simulink model "base_reference"  (R2019a)
settings: Solver=ode23tb  StartTime=0.0  StopTime=60  RelTol=1e-3
model workspace (MAT data in the model file):
  A_mu = 10
  AxlIxx = 62.3745166667
  AxlM = 160
  B_reff = 8.386
  BattCapInit = 26
  BattChargeMax = 32.5
  BattChrgMax = -80000
  BattDischrgMax = 80000
  BattTempBp = [243.1 253.1 263.1 273.1 283.1 298.1 313.1]
  BrkPrsMax = 5000000
  CapLUTBp = [0 0.01 0.02 0.03 0.04 0.05 0.06 0.07 0.08 0.09 0.1 0.11 ... (101 elements, 1x101)]
  CapSOCBp = [0 0.2 0.4 0.6 0.8 1]
  ChrgLmt_bpt = [1 1 1 1 1 1 1 1 0.7 0.35 0]
  Cps = 2
  Cz = 5565.2246438
  CzWhlAxl = 11490.971257
  DCT_Param : struct (value not decoded)
  DLCXref = [0 6 7 14 33.5 34 42 50 60]
  DLCYref = [0 0 -4.5 -4 -3.75 1.5 0.5 0 0]
  D_reff = 0.25826
  DischrgLmt_bpt = [0 0.35 0.7 1 1 1 1 1 1 1 1]
  Downshift_Speeds = [9.5625 12.9375 16.3125 19.6875 23.0625 26.4375 29.8125 33.1875 36.5625 39.9375 43.3125 46.6875 ... (28 elements, 4x7)]
  EV_current = 200
  EV_motion = [20 4 0.8]
  EV_sf = 2000
  Em = [2.8 3.228 3.284 3.361 3.408 3.427 3.472 3.477 3.493 3.504 3.516 3.528 ... (101 elements, 1x101)]
  EngRevLim = 7000
  F0z = [2886 2907]
  F0zWhlAxl = 2907
  Fs = 0
  Fv = 0.0025
  Hmax = 0.25
  Jcomp = 0.0227
  Ki = 251.3274
  Kisa = 346.6583
  Kp_d = 0.47149
  Kp_q = 0.52125
  Ksa = 85.4316
  Ksf = 1996.2651
  Kz = 52451.0065793
  KzWhlAxl = 138031.612078
  Ld = 0.0003752
  Ldq = [0.0003752 0.0004148]
  Lq = 0.0004148
  Mechanical = [0.0227 0.0025 0]
  MotMapEff = 0
  MotSpd = [0 1000 2000 2728.370453 3000 4000 5000 6000 7000 8000 9000 10000]
  MotTrq = [280 280 280 280 254.6479089 190.9859317 152.7887454 127.3239545 109.1348181 95.49296586 84.88263632 76.39437268]
  NCyl = 6
  Ndiff = 7.94
  Np = 2
  Ns = 96
  P = 4
  Pedal_Positions = [0.1 0.4 0.5 0.9]
  PolePairs = 4
  Pstd = 101325
  RInt = [0.008846 0.006389 0.004364 0.002031 0.001443 0.0005603 0.001028 0.009319 0.006554 0.004101 0.002563 0.001825 ... (42 elements, 7x6)]
  Rair = 287
  RegenBrkCutOff = [0 1]
  RegenBrkSpd_bpt = [5 9]
  Rm = 0.15
  Rs = 0.2
  SOC_bpt = [0 10 20 30 40 50 60 70 80 90 100]
  SUS : struct (value not decoded)
  T_eff_bp = [0 20 40 60 80 100 120 140 160 180 200 220 ... (15 elements, 1x15)]
  T_max = 120
  T_mtpa = [0 13.3131834767 26.6278836885 39.9456159322 53.2678926341 66.5962219318 79.9321062746 93.277041051 106.632513247 120.000000141]
  Tc = 0.02
  Trans : struct (value not decoded)
  Tstd = 293.15
  Upshift_Speeds = [12.9375 16.3125 19.6875 33 26.4375 29.8125 33.1875 52.5 39.9375 43.3125 46.6875 77.25 ... (28 elements, 4x7)]
  VEH : struct (value not decoded)
  V_o = 16.7
  V_xlow = 1
  Vd = 0.00346
  WH : struct (value not decoded)
  a = 1.4
  alpha_max = 1.5
  alpha_min = -1.5
  b = 1.8
  ba = 3.4029
  c_zo = 209651
  disk_abore = 0.05
  dt3D = 0.05
  efficiency_table = [85 85 85 85 85 85 85 85 85 85 85 85 ... (180 elements, 12x15)]
  epsilon = 0.1
  f_air = [0 0 0 0 0 0 0 0 0 0 0 0 ... (256 elements, 16x16)]
  f_co = [0 0 0 0 0 0 0 0 0 0 0 0 ... (256 elements, 16x16)]
  f_co2 = [0 0 0 0 0 0 0 0 0 0 0 0 ... (256 elements, 16x16)]
  f_eff = [352.135682859 352.135682859 320.724378192 303.655312657 295.930136708 291.240087194 291.240271258 291.240312459 291.240275452 291.240198499 291.240100781 291.240018769 ... (256 elements, 16x16)]
  f_fuel = [0 0 0 0 0 0 0 0 0 0 0 0 ... (256 elements, 16x16)]
  f_hc = [0 0 0 0 0 0 0 0 0 0 0 0 ... (256 elements, 16x16)]
  f_nox = [0 0 0 0 0 0 0 0 0 0 0 0 ... (256 elements, 16x16)]
  f_pm = [0 0 0 0 0 0 0 0 0 0 0 0 ... (256 elements, 16x16)]
  f_susp_axl_bp = [1 2]
  f_susp_dz_bp = [-0.325022776267 -0.315022776267 -0.305022776267 -0.205022776267 -0.105022776267 -0.00502277626717 0.0949772237328 0.194977223733 0.204977223733 0.214977223733]
  f_susp_dzdot_bp = [-3 -0.3 -0.2 -0.1 0 0.1 0.2 0.3 3]
  f_susp_fmz = [-144070.391448 -93629.24037 -75929.1118915 -20630.5828179 -15385.48216 -10140.3815021 -4895.28084414 349.819813785 -31916.3973792 18437.6709544 -83996.1993354 -33555.0482577 ... (43920 elements, 10x9x61x2x4)]
  f_susp_geom = [0 0 0 0 0 0 0 0 0 0 0 0 ... (3660 elements, 10x61x2x3)]
  f_susp_strgdelta_bp = [-0.523598775598 -0.506145483078 -0.488692190558 -0.471238898038 -0.453785605519 -0.436332312999 -0.418879020479 -0.401425727959 -0.383972435439 -0.366519142919 -0.349065850399 -0.331612557879 ... (61 elements, 1x61)]
  f_tbrake = [0 76.8593923996 105.140482948 131.533638111 157.926793274 176.658631717 176.65727296 176.656856686 176.656879077 176.657093756 176.657404516 176.65772406 ... (256 elements, 16x16)]
  f_tbrake_n_bpt = [0 649.519052838 912.419621844 1175.32019085 1438.22075986 1701.12132886 1964.02189787 2226.92246687 2489.82303588 2752.72360489 3015.62417389 3278.5247429 ... (16 elements, 1x16)]
  f_tbrake_t_bpt = [0 34.6410161514 61.0341713143 87.4273264773 113.82048164 140.213636803 166.606791966 192.999947129 219.393102292 245.786257455 272.179412618 298.572567781 ... (16 elements, 1x16)]
  f_texh = [766.752464599 766.752464599 786.17542386 801.679939032 884.591982581 910.574397722 910.571871054 910.570774534 910.570601632 910.570821151 910.571247242 910.571639815 ... (256 elements, 16x16)]
  f_twc_eff_co = [0.17 0.25 0.45 0.99 0.99 0.99 0.99]
  f_twc_eff_hc = [0.21 0.375 0.75 0.98 0.98 0.98 0.98]
  f_twc_eff_lam = [0.909090909 0.944055944 0.979020979 1 1.013986014 1.048951049 1.083916084]
  f_twc_eff_nox = [0.98 0.98 0.98 0.97 0.05 0.02 0]
  h = 0.134
  id_mtpa = [0 -0.114523352646 -0.457989076459 -1.03008464374 -1.83029075221 -2.85788367342 -4.11193850568 -5.59133329791 -7.29475400168 -9.22070020138]
  idq0 = [0 0]
  idq_limits = [-9.220699542 166.993501392 167.247872355]
  iq_mtpa = [0 18.5827440345 37.1633719111 55.7397734896 74.3098506185 92.871523015 111.422734008 129.961456105 148.485696337 166.993501356]
  lambda_pm = 0.1194
  mechanical = [0.0227 0.0025 0]
  mu_kinetic = 0.35
  numWheel = 4
  num_pads = 2
  omega_init = 0
  path : struct (value not decoded)
  pio = 220000
  power_max = 80000
  q_Fcx = 0
  q_Fz2 = 15.4
  q_Fzy = 0
  q_reo = 0.9974
  q_sx1 = -0.007764
  q_sx10 = 0.2824
  q_sx11 = 5.349
  q_sx12 = 0
  q_sx13 = 0
  q_sx14 = 0
  q_sx2 = 1.1915
  q_sx3 = 0.013948
  q_sx4 = 4.912
  q_sx5 = 1.02
  q_sx6 = 22.83
  q_sx7 = 0.7104
  q_sx8 = -0.023393
  q_sx9 = 0.6581
  q_sy1 = 0.00702
  q_sy2 = 0
  q_sy3 = 0.001515
  q_sy4 = 8.514e-05
  q_sy5 = 0
  q_sy6 = 0
  q_sy7 = 0.9008
  q_sy8 = -0.4089
  q_v1 = 0.0007742
  q_v2 = 0.04667
  r_Bx1 = 12.531
  r_Bx2 = 9.532
  r_Bx3 = 0
  r_By1 = 10.615
  r_By2 = 7.705
  r_By3 = 3.433e-06
  r_By4 = 0
  r_Cx1 = 1.019
  r_Cy1 = 1.0585
  r_Ex1 = -0.4487
  r_Ex2 = -0.4726
  r_Ey1 = 0.3132
  r_Ey2 = 7.63e-06
  r_Hx1 = 0.0002374
  r_Hy1 = 0.011646
  r_Hy2 = 7.63e-06
  r_Vy1 = 0.05654
  r_Vy2 = 7.63e-06
  r_Vy3 = 0
  r_Vy4 = 99.9
  r_Vy5 = 2
  r_Vy6 = 15.814
  r_o = 0.3135
  theta_init = 0
  torque_max = 280
  vehWidth = 2
  w = 1
  w_eff_bp = [0 1000 2000 2728.370453 3000 4000 5000 6000 7000 8000 9000 10000]
values from neighbouring files (symbols this model uses):
  VEH =     [PassVeh14DOF.mat]    (also in model2.mat; model_workspace_reference.mat)
undefined symbols (not defined in the file or in its folder): Disabled, Right
libraries: simulink x8, vehdynlibtire x8, vehdynlibsuspension x7, autolibutils x6, vehdynlibscenariocommon x5, sim3dlib x4, autolibmappedmotor x4, autolibshared x2, sharedtransform x2, vehdynlibviscommon x2, vehdynlibdriver x1, vehdynlibsteering x1
(part 3 of 8)

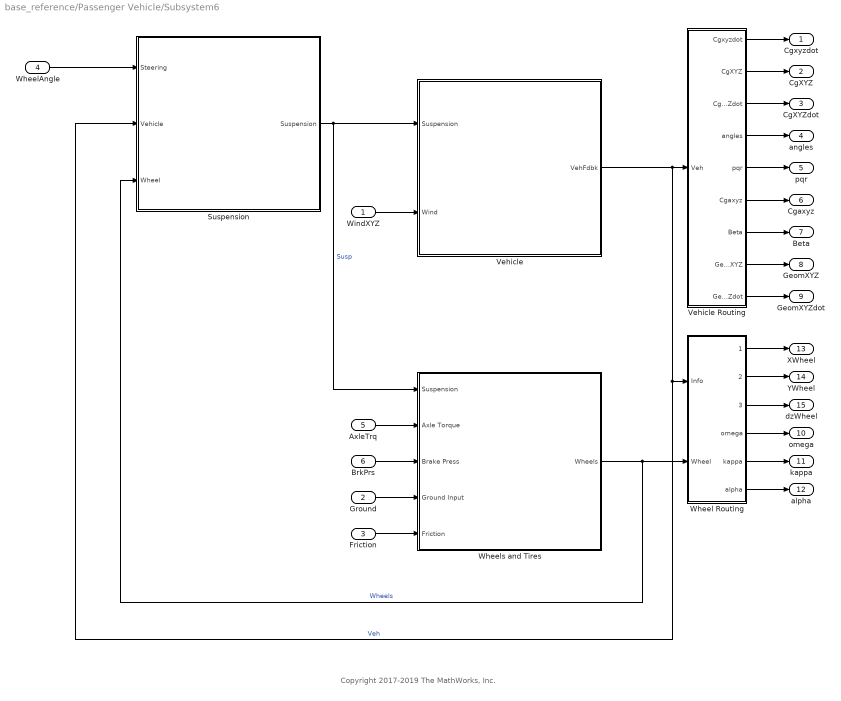
== system base_reference/Passenger Vehicle/Subsystem6 ==
  note: Copyright 2017-2019 The MathWorks, Inc.
  WindXYZ : Inport  Unit=m/s  PortDimensions=3
  Ground : Inport  Port=2  Unit=m  PortDimensions=4
  Friction : Inport  Port=3  Unit=1  PortDimensions=4
  WheelAngle : Inport  Port=4  Unit=rad  PortDimensions=4
  AxleTrq : Inport  Port=5  Unit=N*m  PortDimensions=4
  BrkPrs : Inport  Port=6  PortDimensions=4
  Suspension : Subsystem  VariantControlMode=Label  Variant=on  LabelModeActiveChoice=3
      mask Display:
      | switch str2num(get_param(gcb,'ActiveVariant'))
      |     case 1
      |         image('suspdw.png');
      |     case 2
      |         image([imread('suspindmap.png');imread('suspsamap.png')]);
      |     case 3
      |          image([imread('suspmacp.png');imread('suspsacoil.png')]);
      |     case 4
      |          image('suspmacp.png');
      |     case 5
      |          image('suspindmap.png');
      | end
  Vehicle : Subsystem
      mask Display: image('6dofcar.png');
  Vehicle Routing : Subsystem
  Wheel Routing : Subsystem
  Wheels and Tires : Subsystem
      mask Display: image('wheel3dof.png')
  Cgxyzdot : Outport
  CgXYZ : Outport  Port=2
  CgXYZdot : Outport  Port=3
  angles : Outport  Port=4
  pqr : Outport  Port=5
  Cgaxyz : Outport  Port=6
  Beta : Outport  Port=7
  GeomXYZ : Outport  Port=8
  GeomXYZdot : Outport  Port=9
  omega : Outport  Port=10  PortDimensions=4
  kappa : Outport  Port=11  PortDimensions=4
  alpha : Outport  Port=12  PortDimensions=4
  XWheel : Outport  Port=13
  YWheel : Outport  Port=14
  dzWheel : Outport  Port=15  PortDimensions=4
  wires:
  Vehicle Routing/7(Beta) -> Beta/1
  Vehicle/1(VehFdbk) -> Suspension/2(Vehicle), Wheel Routing/1(Info), Vehicle Routing/1(Veh)  "Veh"
  Friction/1 -> Wheels and Tires/5(Friction)
  WheelAngle/1 -> Suspension/1(Steering)
  WindXYZ/1 -> Vehicle/2(Wind)
  Wheels and Tires/1(Wheels) -> Suspension/3(Wheel), Wheel Routing/2(Wheel)  "Wheels"
  Vehicle Routing/2(CgXYZ) -> CgXYZ/1
  AxleTrq/1 -> Wheels and Tires/2(Axle Torque)
  Vehicle Routing/4(angles) -> angles/1
  Wheel Routing/1(XWheel) -> XWheel/1
  Vehicle Routing/1(Cgxyzdot) -> Cgxyzdot/1
  Wheel Routing/2(YWheel) -> YWheel/1
  Suspension/1(Suspension) -> Wheels and Tires/1(Suspension), Vehicle/1(Suspension)  "Susp"
  Wheel Routing/4(omega) -> omega/1
  Vehicle Routing/6(Cgaxyz) -> Cgaxyz/1
  Vehicle Routing/5(pqr) -> pqr/1
  BrkPrs/1 -> Wheels and Tires/3(Brake Press)
  Vehicle Routing/8(GeomXYZ) -> GeomXYZ/1
  Vehicle Routing/9(GeomXYZdot) -> GeomXYZdot/1
  Ground/1 -> Wheels and Tires/4(Ground Input)
  Wheel Routing/3(ZWheel) -> dzWheel/1
  Wheel Routing/5(kappa) -> kappa/1
  Vehicle Routing/3(CgXYZdot) -> CgXYZdot/1
  Wheel Routing/6(alpha) -> alpha/1

== system base_reference/Reference Generator/3D Engine ==
  note: 1) Add Subsystem or Model blocks as valid variant choices.
      | 2) You cannot connect blocks at this level. At simulation, connectivity is automatically
      | determined, based on the active variant and port name matching.
  VehFdbk : Inport
  3D Engine : Subsystem  VariantControl=1
  3D Engine Disabled : Subsystem  VariantControl=0

== system base_reference/Reference Generator/Reference Generator ==
  "VehFdbk " : Inport
  Constant Radius : Subsystem  AncestorBlock=vehdynlibscenariocommon/Constant Radius  VariantControl=4  mask{t_start=t_start, xdot_r=xdot_r, xdotUnit=mph, R=R, turnDirMask=Right, ay_max=cr_ay_max, ay_stop=off, Parameter6=2}
      mask prompts: t_start "Maneuver start time, t_start [s]:"; xdot_r "Longitudinal velocity reference, xdot_r:"; xdotUnit "Longitudinal velocity reference units, xdotUnit []:"; R "Radius value, R [m]:"; turnDirMask "Turn direction"; ay_max "Lateral acceleration absolute threshold, ay_max [g]:"; ay_stop "Stop simulation at lateral acceleration threshold"
      mask TypeOptions xdotUnit: Longitudinal Velocity Reference/Input Units/Unit
      mask TypeOptions R: Constant Radius/Value
      mask TypeOptions turnDirMask: Constant Radius/turnDirMask
  Double Lane Change : Subsystem  VariantControl=0
  Increasing Steer : Subsystem  VariantControl=1
  Sine with Dwell : Subsystem  VariantControl=3
  Swept Sine : Subsystem  VariantControl=2
  " Vis" : Outport
  " Ref" : Outport  Port=2
  " Fdbk" : Outport  Port=3

== system base_reference/Visualization/ISO 15037-1:2006 ==
  VehFdbk : Inport
  Cntrl : Inport  Port=2
  Disabled : Subsystem  VariantControl=0
  Enabled : Subsystem  VariantControl=1

== system base_reference/Visualization/Scope Type ==
  "VehFdbk " : Inport
  Cntrl : Inport  Port=2
  "Vis " : Inport  Port=3
  DLC : Subsystem  VariantControl=1
  None : Subsystem  VariantControl=0
  XYZ : Subsystem  VariantControl=2
  " Ref" : Outport

== system base_reference/Visualization/Vehicle XY Plotter ==
  "VehFdbk " : Inport
  "Ref " : Inport  Port=2
  XY View : Subsystem  VariantControl=0
  XY View Ref : Subsystem  VariantControl=1

== system base_reference/Controllers/Active Differential Control/No Control ==
  YawRate : Inport
  Steer : Inport  Port=2
  Constant : Constant  Value=0
  Terminator : Terminator
  Terminator1 : Terminator
  Vector Concatenate2 : Concatenate  NumInputs=4
  DiffPrsCmd : Outport
  TrqCmd : Outport  Port=2
  wires:
  Constant/1 -> Vector Concatenate2/1, TrqCmd/1, Vector Concatenate2/4, Vector Concatenate2/3, Vector Concatenate2/2
  Steer/1 -> Terminator1/1
  Vector Concatenate2/1 -> DiffPrsCmd/1  "Reference P"
  YawRate/1 -> Terminator/1

== system base_reference/Controllers/Active Differential Control/Rear Diff Controller ==
  YawRate : Inport
  Steer : Inport  Port=2
  Abs : Abs  ZeroCross=off
  Abs1 : Abs  ZeroCross=off
  Cont LPF : autolibutils/Cont LPF  wc=10*pi  aMode=2
      settings: SourceProductName=Powertrain Blockset  SourceProductBaseCode=PW
  Cont LPF1 : autolibutils/Cont LPF  wc=1*pi  aMode=2
      settings: SourceProductName=Powertrain Blockset  SourceProductBaseCode=PW
  Dead Zone : DeadZone  LowerValue=-.01  UpperValue=.01  ZeroCross=off  SaturateOnIntegerOverflow=on
  Gain : Gain  Gain=1e6
  Gain2 : Gain  Gain=1/4
  Gain3 : Gain  Gain=2e3
  Ground : Ground
  Saturation : Saturate  UpperLimit=0  LowerLimit=-inf  ZeroCross=off
  Saturation1 : Saturate  UpperLimit=inf  LowerLimit=0  ZeroCross=off
  Saturation2 : Saturate  UpperLimit=1e7  LowerLimit=0  ZeroCross=off
  Saturation3 : Saturate  UpperLimit=200  LowerLimit=0  ZeroCross=off
  Subtract : Sum  Inputs=+-
  Vector Concatenate2 : Concatenate  NumInputs=4
  DiffPrsCmd : Outport
  TrqCmd : Outport  Port=2
  wires:
  Vector Concatenate2/1 -> Gain/1  "Reference P"
  Ground/1 -> Vector Concatenate2/2, Vector Concatenate2/1
  Steer/1 -> Gain2/1
  Saturation/1 -> Abs/1
  Saturation1/1 -> Vector Concatenate2/4
  Gain/1 -> Saturation2/1
  Abs/1 -> Vector Concatenate2/3
  Gain3/1 -> Saturation3/1
  Gain2/1 -> Subtract/2
  YawRate/1 -> Subtract/1
  Subtract/1 -> Dead Zone/1
  Abs1/1 -> Gain3/1
  Cont LPF/1 -> Saturation1/1, Saturation/1
  Saturation2/1 -> DiffPrsCmd/1
  Saturation3/1 -> TrqCmd/1
  Dead Zone/1 -> Cont LPF1/1, Cont LPF/1
  Cont LPF1/1 -> Abs1/1

== system base_reference/Controllers/Motor Torque Arbitration and Power Management/Power Management ==
  note: Power Management algorithm:
      | - Estimate Elec power based on mech power using efficiency map
      | - Check if Elec power is within battery power limits
      | - If power within limit , use motor torque command
      | - If power limit exceeded, use limited motor torque
      | - For low Mot Spd, MotPwrReq will be a small number.  Pass through torque command until Mot Spd > 2.
  BattPwrDischrgLmt : Inport
  BattPwrChrgLmt : Inport  Port=2
  MotSpd : Inport  Port=3
  MotTrqCmd : Inport  Port=4
  Abs : Abs
  Check Within Limits : Subsystem
  Compare To Constant : simulink/Logic and Bit Operations/Compare To Constant  relop=<  const=2  OutDataTypeStr=boolean
  ElecToMechPwr : Product  Inputs=*/
  Mech to Elec Power Estimate : Subsystem
  MechPwrToTrq : Product  Inputs=*/
  Switch : Switch  Criteria=u2 > Threshold
  Switch1 : Switch  Criteria=u2 > Threshold
  Torque Limit : Subsystem
  div0protect - poly : autolibutils/div0protect - poly  thresh=2  aMode=aMode
      settings: SourceProductName=Powertrain Blockset  SourceProductBaseCode=PW
  MotTrqCmdFinal : Outport
  wires:
  MotSpd/1 -> Abs/1, Torque Limit/2(MotSpd), div0protect - poly/1, Mech to Elec Power Estimate/2(MotSpd)
  MotTrqCmd/1 -> Switch/1, Switch1/1, Mech to Elec Power Estimate/1(MotTrqCmd)
  div0protect - poly/1 -> MechPwrToTrq/2
  Mech to Elec Power Estimate/2(Eff2k) -> ElecToMechPwr/2
  ElecToMechPwr/1 -> MechPwrToTrq/1
  MechPwrToTrq/1 -> Switch/3
  Torque Limit/1(MotTrqCmd) -> MotTrqCmdFinal/1
  BattPwrDischrgLmt/1 -> Check Within Limits/1(up)
  Mech to Elec Power Estimate/1(MotPwrElecReq) -> Check Within Limits/2(u)
  BattPwrChrgLmt/1 -> Check Within Limits/3(lo)
  Check Within Limits/2(y) -> ElecToMechPwr/1
  Switch/1 -> Switch1/3
  Check Within Limits/1(InLimit) -> Switch/2
  Switch1/1 -> Torque Limit/1(MotTrq)
  Abs/1 -> Compare To Constant/1
  Compare To Constant/1 -> Switch1/2

== system base_reference/Controllers/Regen Braking Control/Parallel Regen Braking ==
  VehSpd : Inport
  MotSpd : Inport  Port=2
  "BrkPrsReq " : Inport  Port=3
  BattSoc : Inport  Port=4
  ChrgLmt : Lookup_n-D  NumberOfTableDimensions=1  BreakpointsForDimension1=[0:10:100]  Table=[1 1 1 1 1 1 1 1 0.7 0.35 0]  ExtrapMethod=Clip  UseLastTableValue=on  InternalRulePriority=Speed  RndMeth=Simplest  InputSameDT=on
  Gain : Gain  Gain=-1
  MaxMotorTrqVsSpd : Lookup_n-D  NumberOfTableDimensions=1  BreakpointsForDimension1=MotSpd  Table=MotTrq  ExtrapMethod=Clip  UseLastTableValue=on  InternalRulePriority=Speed  OutDataTypeStr=Inherit: Inherit from 'Table data'  RndMeth=Simplest  InputSameDT=on
  Product1 : Product
  Product3 : Product
  RegenBrakingCutoff : Lookup_n-D  NumberOfTableDimensions=1  BreakpointsForDimension1=[2.2 4.5]  Table=[0 1]  ExtrapMethod=Clip  UseLastTableValue=on  InternalRulePriority=Speed  RndMeth=Simplest  InputSameDT=on
  rads_to_rpm : Gain  Gain=30/pi
  " MotTrqCmdRegen" : Outport
  " BrkCmd" : Outport  Port=2
  wires:
  Gain/1 -> " MotTrqCmdRegen"/1
  BattSoc/1 -> ChrgLmt/1
  Product3/1 -> Gain/1  "MotTrqRegen"
  Product1/1 -> Product3/2  "RegenFactor"
  RegenBrakingCutoff/1 -> Product1/1
  VehSpd/1 -> RegenBrakingCutoff/1
  ChrgLmt/1 -> Product1/2
  MaxMotorTrqVsSpd/1 -> Product3/1  "MotTrqMax"
  rads_to_rpm/1 -> MaxMotorTrqVsSpd/1
  MotSpd/1 -> rads_to_rpm/1
  "BrkPrsReq "/1 -> " BrkCmd"/1  "BrkPrsReq"

== system base_reference/Controllers/Regen Braking Control/Series Regen Braking ==
  note: - Total brake torque request based on brake pressure and parameters of disc brakes
      | - Use as much regenerative motor braking as possible
      | - Any braking torque request that cannot be provided by the motor, will be provided by the friction brakes
  note: T / 4 brakes*(muk*pi*Ba^2*Rm*Npads/4)
  note: 4 brakes*(muk*pi*Ba^2*Rm*Npads/4)*P
  VehSpd : Inport
  MotSpd : Inport  Port=2
  "BrkPrsReq " : Inport  Port=3
  BattSoc : Inport  Port=4
  ChrgLmt : Lookup_n-D  NumberOfTableDimensions=1  BreakpointsForDimension1=SOC_bpt  Table=ChrgLmt_bpt  ExtrapMethod=Clip  UseLastTableValue=on  InternalRulePriority=Speed  RndMeth=Simplest  InputSameDT=on
  Constant : Constant  Value=4*(mu_kinetic*pi*disk_abore^2*Rm*num_pads/4)
  Constant1 : Constant  Value=4*(mu_kinetic*pi*disk_abore^2*Rm*num_pads/4)
  Gain : Gain  Gain=-1
  MaxMotTrqVsSpd : Lookup_n-D  NumberOfTableDimensions=1  BreakpointsForDimension1=MotSpd  Table=MotTrq  ExtrapMethod=Clip  UseLastTableValue=on  InternalRulePriority=Speed  OutDataTypeStr=Inherit: Inherit from 'Table data'  RndMeth=Simplest  InputSameDT=on
  MinMax : MinMax  Inputs=2
  MotTrqReflectedToWheels : Gain  Gain=Ndiff
  Negative 5 : Saturate  UpperLimit=inf  LowerLimit=0
  Product1 : Product
  Product2 : Product
  Product3 : Product
  Product4 : Product  Inputs=*/
  RegenBrakingCutoff : Lookup_n-D  NumberOfTableDimensions=1  BreakpointsForDimension1=RegenBrkSpd_bpt  Table=RegenBrkCutOff  ExtrapMethod=Clip  UseLastTableValue=on  InternalRulePriority=Speed  RndMeth=Simplest  InputSameDT=on
  Subtract : Sum  Inputs=+-
  WhlTrqReflectedToMot : Gain  Gain=1/Ndiff
  rads_to_rpm : Gain  Gain=30/pi
  " MotTrqCmdRegen" : Outport
  " BrkCmd" : Outport  Port=2
  wires:
  Product3/1 -> WhlTrqReflectedToMot/1, Subtract/2  "MotTrqRegenWhl"
  Product4/1 -> " BrkCmd"/1
  Constant1/1 -> Product4/2
  Constant/1 -> Product2/2
  "BrkPrsReq "/1 -> Product2/1  "BrkPrsReq"
  rads_to_rpm/1 -> MaxMotTrqVsSpd/1
  MaxMotTrqVsSpd/1 -> MotTrqReflectedToWheels/1  "MotTrqMax"
  Product2/1 -> MinMax/1, Subtract/1  "BrkTrqReqTotal"
  MinMax/1 -> Product3/1  "min"
  ChrgLmt/1 -> Product1/2
  VehSpd/1 -> RegenBrakingCutoff/1
  RegenBrakingCutoff/1 -> Product1/1
  Product1/1 -> Product3/2  "RegenFactor"
  Subtract/1 -> Negative 5/1
  BattSoc/1 -> ChrgLmt/1
  Negative 5/1 -> Product4/1  "BrkTrqFric"
  MotSpd/1 -> rads_to_rpm/1
  MotTrqReflectedToWheels/1 -> MinMax/2  "MotTrqMaxWhls"
  WhlTrqReflectedToMot/1 -> Gain/1
  Gain/1 -> " MotTrqCmdRegen"/1  "MotTrqCmdRegen"

== system base_reference/Driver Commands/Driver Commands/Longitudinal Driver ==
  VehRef : Inport
  VehFdbk : Inport  Port=2
  Bus Creator1 : BusCreator  Inputs=4
  Bus Selector : BusSelector  OutputSignals=Body.xdot
  Bus Selector1 : BusSelector  OutputSignals=Steer,LngRef
  Dead Zone : DeadZone  LowerValue=-.1  UpperValue=.1  SaturateOnIntegerOverflow=on
  Ground : Ground
  Longitudinal Driver : autolibshared/Longitudinal Driver  cntrlType=Predictive  shftType=None  velUnits=m/s  gearOut=on  Kp=5  Ki=5  Kff=.1  Kg=0  VehVelVec=[0 100]  KffVec=[.1 .1]  KpVec=[10 10]  KiVec=[5 5]  KgVec=[0 0]  m=VEH.Mass  Kpt=3000  tau=.5  L=3  aR=200  bR=2.5  cR=.5  g=9.81  vnom=5  Kaw=1  tauerr=.1  tauPt=2  GearInit=0  tShift=.1  pdlVec=[0.1 0.4 0.5 0.9]  upShftTbl=[-1 12.9375 26.4375 39.9375 51.18749999999999 62.4375 72.84375 83.25;-1 16.3125 29.8125 43.3125 54.5624 65.8125 76.78125 87.75;-1 19.6875 33.1875 46.68749999999999 57.9375 69.1875 80.71875 92.25;-1 33 52.5 77.25 100.5 138.75 161.875 185]  dwnShftTbl=[1 9.5625 23.0625 36.5625 47.8125 59.0625 68.90625 78.75;1 12.9375 26.4375 39.9375 51.18749999999999 62.4375 72.84375 83.25;1 16.3125 29.8125 43.3125 54.562499 65.8125 76.78125 87.75;1 19.6875 33.1875 46.68749999999999 57.9375 69.1875 80.71875 92.25]  tClutch=.5  tRev=.5  tPark=120  aMode=2  UpGearVec="[0  1  2  3  4  5  6  7]"  DownGearVec="[1  2  3  4  5  6  7  8]"
      settings: SourceProductName=Powertrain Blockset  SourceProductBaseCode=PW
  Terminator3 : Terminator
  Unit Conversion : UnitConversion
  Driver : Outport
  wires:
  Dead Zone/1 -> Longitudinal Driver/2
  Bus Creator1/1 -> Driver/1
  Unit Conversion/1 -> Bus Creator1/1  "Steer"
  Longitudinal Driver/3 -> Bus Creator1/3  "Brake"
  Longitudinal Driver/1 -> Terminator3/1
  Bus Selector1/2 -> Longitudinal Driver/1  "<LngRef>"
  VehRef/1 -> Bus Selector1/1
  VehFdbk/1 -> Bus Selector/1
  Bus Selector/1 -> Dead Zone/1  "<xdot>"
  Longitudinal Driver/2 -> Bus Creator1/2  "Accel"
  Ground/1 -> Longitudinal Driver/3
  Longitudinal Driver/4 -> Bus Creator1/4  "Gear"
  Bus Selector1/1 -> Unit Conversion/1  "<Steer>"

== system base_reference/Driver Commands/Driver Commands/Open Loop Constant Radius ==
  VehFdbk : Inport
  SteerCmd : Inport  Port=2
  Accel : Inport  Port=3
  Brake : Inport  Port=4
  Gear : Inport  Port=5
  Bus Creator1 : BusCreator  Inputs=4
  Terminator : Terminator
  Unit Conversion{,1..3} (4 alike) : UnitConversion
  Wheel Angle Limit * Steer Ratio : Gain  Gain=40*pi/180*18
  Driver : Outport
  wires:
  Unit Conversion3/1 -> Bus Creator1/4  "Gear"
  Unit Conversion2/1 -> Bus Creator1/3  "Brake"
  Wheel Angle Limit * Steer Ratio/1 -> Bus Creator1/1  "Steer"
  Bus Creator1/1 -> Driver/1
  Unit Conversion/1 -> Wheel Angle Limit * Steer Ratio/1  "SteerCmd"
  Accel/1 -> Unit Conversion1/1
  VehFdbk/1 -> Terminator/1
  SteerCmd/1 -> Unit Conversion/1
  Unit Conversion1/1 -> Bus Creator1/2  "Accel"
  Brake/1 -> Unit Conversion2/1
  Gear/1 -> Unit Conversion3/1

== system base_reference/Driver Commands/Driver Commands/Predictive Driver ==
  VehRef : Inport
  VehFdbk : Inport  Port=2
  Bus Creator1 : BusCreator  Inputs=4
  Bus Selector : BusSelector  OutputSignals=Body.xdot,Body.Y,Body.ydot,Body.psi,Body.r
  Bus Selector1 : BusSelector  OutputSignals=LngRef,LtrlRef,ThrotKill
  Constant : Constant  Value=0
  Dead Zone : DeadZone  LowerValue=-.5  UpperValue=.5  ZeroCross=off  SaturateOnIntegerOverflow=on
  Dead Zone1 : DeadZone  LowerValue=-1e-2  UpperValue=1e-2  ZeroCross=off  SaturateOnIntegerOverflow=on
  Ground : Ground
  Linear Predictive Driver : vehdynlibdriver/Predictive Driver  cntrlType=Predictive  shftType=Reverse, Neutral, Drive  velUnits=m/s  gearOut=on  Kp=3  Ki=1  Kff=1  Kg=0  VehVelVec=[0 100]  KffVec=[.1 .1]  KpVec=[10 10]  KiVec=[5 5]  KgVec=[0 0]  vnom=5  Kaw=1  tauerr=.075  a=VEH.FrontAxlePositionfromCG  b=VEH.RearAxlePositionfromCG  m=VEH.Mass  I=VEH.YawMomentInertia  Cy_f=5000  Cy_r=7000  theta=40*pi/180  tau=0.03  L=1.0  Kpt=20000  aR=200  bR=2.5  cR=.5  g=9.81  GearInit=0  tShift=.1  pdlVec=[0.1 0.4 0.5 0.9]  upShftTbl=[-1 12.9375 26.4375 39.9375 51.18749999999999 62.4375 72.84375 83.25;-1 16.3125 29.8125 43.3125 54.5624 65.8125 76.78125 87.75;-1 19.6875 33.1875 46.68749999999999 57.9375 69.1875 80.71875 92.25;-1 33 52.5 77.25 100.5 138.75 161.875 185]  dwnShftTbl=[-1 12.9375 26.4375 39.9375 51.18749999999999 62.4375 72.84375 83.25;-1 16.3125 29.8125 43.3125 54.5624 65.8125 76.78125 87.75;-1 19.6875 33.1875 46.68749999999999 57.9375 69.1875 80.71875 92.25;-1 33 52.5 77.25 100.5 138.75 161.875 185]  tClutch=.5  tRev=.5  tPark=120  aMode=2  UpGearVec="[0  1  2  3  4  5  6  7]"  DownGearVec="[1  2  3  4  5  6  7  8]"
      link override Shift: LabelModeActiveChoice=0
      settings: SourceProductName=Vehicle Dynamics Blockset  SourceProductBaseCode=VE
  Switch : Switch  Criteria=u2 > Threshold
  Terminator : Terminator
  Wheel Angle Limit * Steer Ratio : Gain  Gain=20*pi/180*18
  Driver : Outport
  wires:
  Switch/1 -> Bus Creator1/2  "Accel"
  Linear Predictive Driver/2 -> Dead Zone1/1  "SteerCmd"
  Linear Predictive Driver/3 -> Switch/3  "AccelCmd"
  Bus Selector/3 -> Linear Predictive Driver/6  "<ydot>"
  Ground/1 -> Linear Predictive Driver/3
  Constant/1 -> Switch/1
  Bus Selector/1 -> Dead Zone/1  "<xdot>"
  Bus Selector/2 -> Linear Predictive Driver/5  "<Y>"
  Bus Selector1/3 -> Switch/2  "<ThrotKill>"
  Bus Creator1/1 -> Driver/1
  Dead Zone/1 -> Linear Predictive Driver/4
  Linear Predictive Driver/1 -> Terminator/1
  Bus Selector/4 -> Linear Predictive Driver/7  "<psi>"
  VehFdbk/1 -> Bus Selector/1
  Bus Selector1/2 -> Linear Predictive Driver/2  "<LtrlRef>"
  Bus Selector/5 -> Linear Predictive Driver/8  "<r>"
  Dead Zone1/1 -> Wheel Angle Limit * Steer Ratio/1
  VehRef/1 -> Bus Selector1/1
  Bus Selector1/1 -> Linear Predictive Driver/1  "<LngRef>"
  Wheel Angle Limit * Steer Ratio/1 -> Bus Creator1/1  "Steer"
  Linear Predictive Driver/4 -> Bus Creator1/3  "Brake"
  Linear Predictive Driver/5 -> Bus Creator1/4  "Gear"

== system base_reference/Environment/Ground Feedback/3D Engine ==
  Friction : Inport
  Bus Creator : BusCreator  Inputs=4
  Bus Creator2 : BusCreator  Inputs=4
  Bus Creator3 : BusCreator  Inputs=2
  Bus Selector : BusSelector  OutputSignals=HitLoc
  Data Type Conversion : DataTypeConversion
  Demux : Demux
  Demux1 : Demux
  Passenger Vehicle Ray Trace Set : sim3dlib/Vehicle Terrain Sensor  ActorTag=SimulinkVehicle1  VehExtEn=Constant  TireRadiiExt=Constant  VehCntrLngthVal=0  TireRadiiVal=0  VehRayLngth=10  LfRayLngth=20  RfRayLngth=20  LrRayLngth=20  RrRayLngth=20  VehRayOffset=0  LfRayOffset=-1  RfRayOffset=-1  LrRayOffset=-1  RrRayOffset=-1  VehEn=on  LfEn=on  RfEn=on  LrEn=on  RrEn=on  DbgEn=off  Ts=.03  aMode=aMode
      settings: SourceProductName=Vehicle Dynamics Blockset  SourceProductBaseCode=VE
  Rate Transition : RateTransition
  Reshape10 : Reshape  OutputDimensionality=Row vector (2-D)
  Selector1 : Selector  InputPortWidth=5  IndexOptions=Index vector (dialog)  Indices=[2:5]  OutputSizes=1
  Signal Specification : SignalSpecification  Unit=m
  Signal Specification1 : SignalSpecification  Unit=1
  Terminator1 : Terminator
  Terminator2 : Terminator
  Zend Select : Selector  NumberOfDimensions=2  InputPortWidth=3  IndexOptions=Select all,Index vector (dialog)  Indices=[1 3],3  OutputSizes=1,1
  Ground : Outport
  wires:
  Selector1/1 -> Rate Transition/1
  Zend Select/1 -> Reshape10/1
  Bus Selector/1 -> Zend Select/1  "<HitLoc>"
  Passenger Vehicle Ray Trace Set/2 -> Terminator1/1
  Passenger Vehicle Ray Trace Set/3 -> Terminator2/1
  Reshape10/1 -> Selector1/1
  Passenger Vehicle Ray Trace Set/1 -> Bus Selector/1
  Rate Transition/1 -> Data Type Conversion/1
  Demux/2 -> Bus Creator/2  "G_FR_z"
  Demux/1 -> Bus Creator/1  "G_FL_z"
  Demux/4 -> Bus Creator/4  "G_RR_z"
  Demux/3 -> Bus Creator/3  "G_RL_z"
  Signal Specification/1 -> Demux/1
  Signal Specification1/1 -> Demux1/1
  Demux1/1 -> Bus Creator2/1  "mu_FL"
  Bus Creator/1 -> Bus Creator3/1  "z"
  Demux1/3 -> Bus Creator2/3  "mu_RL"
  Demux1/4 -> Bus Creator2/4  "mu_RR"
  Demux1/2 -> Bus Creator2/2  "mu_FR"
  Bus Creator2/1 -> Bus Creator3/2  "mu"
  Bus Creator3/1 -> Ground/1
  Friction/1 -> Signal Specification1/1
  Data Type Conversion/1 -> Signal Specification/1

== system base_reference/Environment/Ground Feedback/Constant ==
  Friction : Inport
  Bus Creator : BusCreator  Inputs=4
  Bus Creator2 : BusCreator  Inputs=4
  Bus Creator3 : BusCreator  Inputs=2
  Constant1 : Constant  Value=zeros(4,1)
  Demux : Demux
  Demux1 : Demux
  Signal Specification : SignalSpecification  Unit=m
  Signal Specification1 : SignalSpecification  Unit=1
  Ground : Outport
  wires:
  Constant1/1 -> Signal Specification/1
  Signal Specification/1 -> Demux/1
  Demux/4 -> Bus Creator/4  "G_RR_z"
  Demux/1 -> Bus Creator/1  "G_FL_z"
  Demux/3 -> Bus Creator/3  "G_RL_z"
  Demux/2 -> Bus Creator/2  "G_FR_z"
  Bus Creator/1 -> Bus Creator3/1  "z"
  Demux1/3 -> Bus Creator2/3  "mu_RL"
  Demux1/4 -> Bus Creator2/4  "mu_RR"
  Demux1/1 -> Bus Creator2/1  "mu_FL"
  Demux1/2 -> Bus Creator2/2  "mu_FR"
  Bus Creator2/1 -> Bus Creator3/2  "mu"
  Friction/1 -> Signal Specification1/1
  Signal Specification1/1 -> Demux1/1
  Bus Creator3/1 -> Ground/1

== system base_reference/Passenger Vehicle/Subsystem5/Brake Hydraulics1 ==
  BrkPrsCmd : Inport
  Circuit : Switch  Criteria=u2 ~= 0
  Constant : Constant  Value=-1
  Gain4 : Gain  Gain=8e6
  Valve : autolibutils/Cont LPF  wc=200*2*pi  aMode=2
      settings: SourceProductName=Powertrain Blockset  SourceProductBaseCode=PW
  Volume : Integrator  LimitOutput=on  UpperSaturationLimit=1  LowerSaturationLimit=0  AbsoluteTolerance=1e-3
  BrkPrs : Outport
  wires:
  Volume/1 -> Gain4/1
  Valve/1 -> Volume/1  "Flow"
  BrkPrsCmd/1 -> Circuit/1, Circuit/2
  Gain4/1 -> BrkPrs/1  "Pressure"
  Circuit/1 -> Valve/1
  Constant/1 -> Circuit/3

== system base_reference/Passenger Vehicle/Subsystem6/Suspension ==
  Steering : Inport
  Vehicle : Inport  Port=2
  Wheel : Inport  Port=3
  Double Wishbone Suspension : Subsystem  VariantControl=1
      mask Display: image('suspdw.png');
  Independent Mapped Front Suspension Mapped Solid Axle Rear Suspension : Subsystem  VariantControl=2
      mask Display: image([imread('suspindmap.png');imread('suspsamap.png')]);
  MacPherson Front Suspension Solid Axle Rear Suspension : Subsystem  VariantControl=3
      mask Display: image([imread('suspmacp.png');imread('suspsacoil.png')]);
  MacPherson Suspension : Subsystem  VariantControl=4
      mask Display: image('suspmacp.png');
  Mapped Suspension : Subsystem  VariantControl=5
      mask Display: image('suspindmap.png');
  Suspension : Outport

== system base_reference/Passenger Vehicle/Subsystem6/Vehicle ==
  Suspension : Inport
  Wind : Inport  Port=2
  Variant Subsystem : Subsystem  VariantControlMode=Label  Variant=on  LabelModeActiveChoice=1
  VehFdbk : Outport
  wires:
  Variant Subsystem/1(VehFdbk) -> VehFdbk/1  "VehFdbk"
  Wind/1 -> Variant Subsystem/2(Wind)
  Suspension/1 -> Variant Subsystem/1(Suspension)

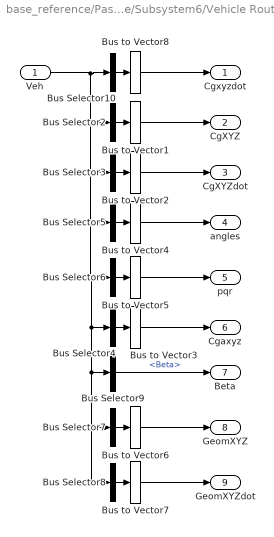
== system base_reference/Passenger Vehicle/Subsystem6/Vehicle Routing ==
  Veh : Inport
  Bus Selector10 : BusSelector  OutputSignals=BdyFrm.Cg.Vel.xdot,BdyFrm.Cg.Vel.ydot,BdyFrm.Cg.Vel.zdot  OutputAsBus=on
  Bus Selector2 : BusSelector  OutputSignals=InertFrm.Cg.Disp.X,InertFrm.Cg.Disp.Y,InertFrm.Cg.Disp.Z  OutputAsBus=on
  Bus Selector3 : BusSelector  OutputSignals=InertFrm.Cg.Vel.Xdot,InertFrm.Cg.Vel.Ydot,InertFrm.Cg.Vel.Zdot  OutputAsBus=on
  Bus Selector4 : BusSelector  OutputSignals=BdyFrm.Cg.Acc.ax,BdyFrm.Cg.Acc.ay,BdyFrm.Cg.Acc.az  OutputAsBus=on
  Bus Selector5 : BusSelector  OutputSignals=InertFrm.Cg.Ang.phi,InertFrm.Cg.Ang.theta,InertFrm.Cg.Ang.psi  OutputAsBus=on
  Bus Selector6 : BusSelector  OutputSignals=BdyFrm.Cg.AngVel.p,BdyFrm.Cg.AngVel.q,BdyFrm.Cg.AngVel.r  OutputAsBus=on
  Bus Selector7 : BusSelector  OutputSignals=InertFrm.Geom.Disp.X,InertFrm.Geom.Disp.Y,InertFrm.Geom.Disp.Z  OutputAsBus=on
  Bus Selector8 : BusSelector  OutputSignals=InertFrm.Geom.Vel.Xdot,InertFrm.Geom.Vel.Ydot,InertFrm.Geom.Vel.Zdot  OutputAsBus=on
  Bus Selector9 : BusSelector  OutputSignals=BdyFrm.Geom.Ang.Beta
  Bus to Vector{1..8} (8 alike) : BusToVector
  Cgxyzdot : Outport
  CgXYZ : Outport  Port=2
  CgXYZdot : Outport  Port=3
  angles : Outport  Port=4
  pqr : Outport  Port=5
  Cgaxyz : Outport  Port=6
  Beta : Outport  Port=7
  GeomXYZ : Outport  Port=8
  GeomXYZdot : Outport  Port=9
  wires:
  Bus Selector3/1 -> Bus to Vector2/1
  Bus to Vector1/1 -> CgXYZ/1
  Bus to Vector5/1 -> pqr/1
  Bus Selector5/1 -> Bus to Vector4/1
  Bus Selector6/1 -> Bus to Vector5/1
  Bus to Vector4/1 -> angles/1
  Bus to Vector8/1 -> Cgxyzdot/1
  Bus Selector2/1 -> Bus to Vector1/1
  Bus Selector8/1 -> Bus to Vector7/1
  Bus to Vector6/1 -> GeomXYZ/1
  Bus Selector9/1 -> Beta/1  "<Beta>"
  Bus Selector4/1 -> Bus to Vector3/1
  Bus Selector10/1 -> Bus to Vector8/1
  Bus to Vector7/1 -> GeomXYZdot/1
  Bus to Vector3/1 -> Cgaxyz/1
  Bus Selector7/1 -> Bus to Vector6/1
  Bus to Vector2/1 -> CgXYZdot/1
  Veh/1 -> Bus Selector8/1, Bus Selector7/1, Bus Selector9/1, Bus Selector4/1, Bus Selector6/1, Bus Selector5/1, Bus Selector3/1, Bus Selector2/1, Bus Selector10/1

== system base_reference/Passenger Vehicle/Subsystem6/Wheel Routing ==
  Info : Inport
  Wheel : Inport  Port=2
  Bus Selector : BusSelector  OutputSignals=InertFrm.FrntAxl.Lft.Disp.Y,InertFrm.FrntAxl.Rght.Disp.Y,InertFrm.RearAxl.Lft.Disp.Y,InertFrm.RearAxl.Rght.Disp.Y
  Bus Selector1 : BusSelector  OutputSignals=InertFrm.FrntAxl.Lft.Disp.X,InertFrm.FrntAxl.Rght.Disp.X,InertFrm.RearAxl.Lft.Disp.X,InertFrm.RearAxl.Rght.Disp.X
  Bus Selector2 : BusSelector  OutputSignals=TireFrame.z,TireFrame.omega,TireFrame.Kappa,TireFrame.Alpha
  Bus Selector3 : BusSelector  OutputSignals=InertFrm.FrntAxl.Lft.Disp.Z,InertFrm.FrntAxl.Rght.Disp.Z,InertFrm.RearAxl.Lft.Disp.Z,InertFrm.RearAxl.Rght.Disp.Z
  Bus Selector4 : BusSelector  OutputSignals=BdyFrm.FrntAxl.Lft.Disp.z,BdyFrm.FrntAxl.Rght.Disp.z,BdyFrm.RearAxl.Lft.Disp.z,BdyFrm.RearAxl.Rght.Disp.z
  Subtract : Sum  Inputs=-+-
  Vector Concatenate{1..4} (4 alike) : Concatenate  NumInputs=4
  XWheel : Outport  Unit=m
  YWheel : Outport  Port=2  Unit=m
  ZWheel : Outport  Port=3  PortDimensions=4
  omega : Outport  Port=4  PortDimensions=4
  kappa : Outport  Port=5  PortDimensions=4
  alpha : Outport  Port=6  PortDimensions=4
  wires:
  Bus Selector1/4 -> Vector Concatenate2/4  "<X>"
  Bus Selector/1 -> Vector Concatenate1/1  "<Y>"
  Bus Selector1/3 -> Vector Concatenate2/3  "<X>"
  Bus Selector/4 -> Vector Concatenate1/4  "<Y>"
  Bus Selector1/2 -> Vector Concatenate2/2  "<X>"
  Bus Selector/3 -> Vector Concatenate1/3  "<Y>"
  Bus Selector/2 -> Vector Concatenate1/2  "<Y>"
  Vector Concatenate1/1 -> YWheel/1
  Bus Selector1/1 -> Vector Concatenate2/1  "<X>"
  Vector Concatenate2/1 -> XWheel/1
  Bus Selector2/1 -> Subtract/3  "<z>"
  Bus Selector2/2 -> omega/1  "<omega>"
  Bus Selector2/3 -> kappa/1  "<Kappa>"
  Bus Selector2/4 -> alpha/1  "<Alpha>"
  Wheel/1 -> Bus Selector2/1
  Subtract/1 -> ZWheel/1
  Info/1 -> Bus Selector1/1, Bus Selector4/1, Bus Selector3/1, Bus Selector/1
  Bus Selector3/2 -> Vector Concatenate3/2  "<Z>"
  Bus Selector3/3 -> Vector Concatenate3/3  "<Z>"
  Bus Selector3/4 -> Vector Concatenate3/4  "<Z>"
  Bus Selector3/1 -> Vector Concatenate3/1  "<Z>"
  Vector Concatenate3/1 -> Subtract/2
  Vector Concatenate4/1 -> Subtract/1
  Bus Selector4/1 -> Vector Concatenate4/1  "<z>"
  Bus Selector4/4 -> Vector Concatenate4/4  "<z>"
  Bus Selector4/3 -> Vector Concatenate4/3  "<z>"
  Bus Selector4/2 -> Vector Concatenate4/2  "<z>"

== system base_reference/Passenger Vehicle/Subsystem6/Wheels and Tires ==
  Suspension : Inport
  Axle Torque : Inport  Port=2
  Brake Press : Inport  Port=3  Unit=Pa
  Ground Input : Inport  Port=4
  Friction : Inport  Port=5  PortDimensions=4
  Bus Selector1 : BusSelector  OutputSignals=Whl.Ang,Whl.F,Whl.AngVel,Whl.xdot,Whl.ydot
  Constant3 : Constant  Value=zeros(4,1)
  Cont LPF : autolibutils/Cont LPF  wc=100*2*pi  aMode=2
      settings: SourceProductName=Powertrain Blockset  SourceProductBaseCode=PW
  Cont LPF1 : autolibutils/Cont LPF  wc=100*2*pi  aMode=2
      settings: SourceProductName=Powertrain Blockset  SourceProductBaseCode=PW
  Manual Switch6 : ManualSwitch
  Matrix Concatenate : Concatenate  NumInputs=3  Mode=Multidimensional array
  Reshape1 : Reshape
  Reshape2 : Reshape
  Saturation : Saturate  UpperLimit=inf  LowerLimit=-10*9.81*2000  ZeroCross=off
  Selector : Selector  NumberOfDimensions=2  InputPortWidth=3  IndexOptions=Index vector (dialog),Select all  Indices=[3],1  OutputSizes=1,1
  Selector1 : Selector  NumberOfDimensions=2  InputPortWidth=1  IndexOptions=Index vector (dialog),Select all  Indices=[3],1  OutputSizes=1,1
  Selector2 : Selector  NumberOfDimensions=2  InputPortWidth=3  IndexOptions=Index vector (dialog),Select all  Indices=3,1  OutputSizes=1,1
  Selector3 : Selector  NumberOfDimensions=2  InputPortWidth=3  IndexOptions=Index vector (dialog),Select all  Indices=1,1  OutputSizes=1,1
  Terminator{,1,3..5} (5 alike) : Terminator
  VDBS : Subsystem  VariantControl=0
  Wheels : Outport
  wires:
  VDBS/1(Wheels) -> Wheels/1  "Wheels"
  Bus Selector1/2 -> Selector/1  "<F>"
  VDBS/2(FrntAxlF) -> Terminator/1
  VDBS/3(RearAxlF) -> Terminator1/1
  VDBS/4(omega) -> Terminator3/1
  VDBS/5(SteerTrq) -> Terminator4/1
  Selector1/1 -> Reshape1/1
  Matrix Concatenate/1 -> VDBS/7(VehVel)
  Axle Torque/1 -> VDBS/3(AxleTrq)
  Selector2/1 -> VDBS/1(WheelAng)  "Wheel Angles"
  Constant3/1 -> Manual Switch6/1
  Manual Switch6/1 -> VDBS/2(CamberAng)  "Camber Angles"
  Selector/1 -> Reshape2/1
  Saturation/1 -> VDBS/5(Fz)
  Ground Input/1 -> VDBS/8(Ground Level)
  VDBS/7(SuspWhlVz) -> Matrix Concatenate/3  "zdot"
  Bus Selector1/1 -> Cont LPF1/1  "<Ang>"
  Selector3/1 -> Manual Switch6/2  "Camber Angles"
  Suspension/1 -> Bus Selector1/1
  Bus Selector1/4 -> Matrix Concatenate/1  "<xdot>"
  Bus Selector1/5 -> Matrix Concatenate/2  "<ydot>"
  VDBS/6(SuspWhlPz) -> Terminator5/1  "z"
  Reshape2/1 -> Cont LPF/1
  Bus Selector1/3 -> Selector1/1  "<AngVel>"
  Reshape1/1 -> VDBS/6(r)
  Brake Press/1 -> VDBS/4(BrkPrs)
  Friction/1 -> VDBS/9(Friction)
  Cont LPF/1 -> Saturation/1
  Cont LPF1/1 -> Selector3/1, Selector2/1

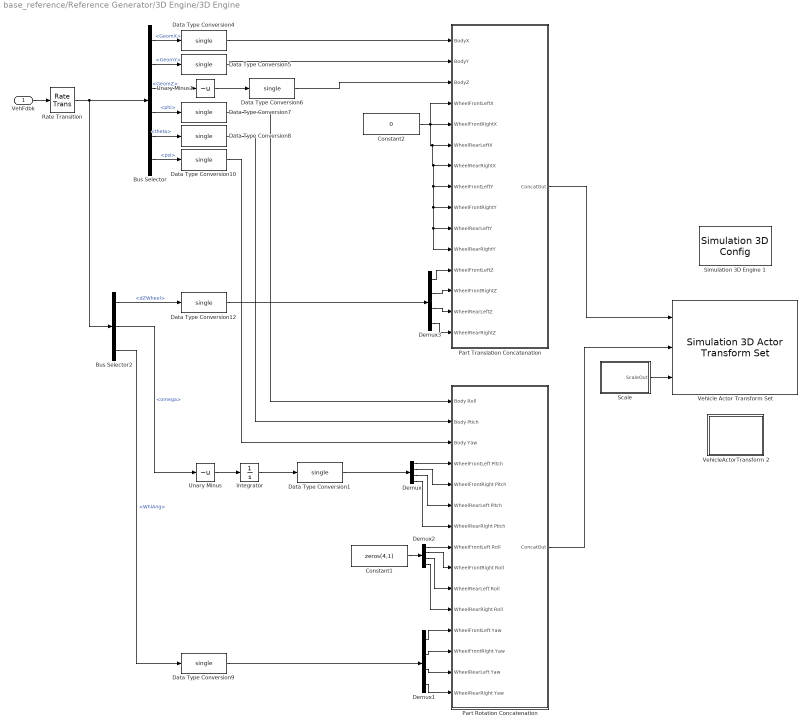
== system base_reference/Reference Generator/3D Engine/3D Engine ==
  VehFdbk : Inport
  Bus Selector : BusSelector  OutputSignals=Body.GeomX,Body.GeomY,Body.GeomZ,Body.phi,Body.theta,Body.psi
  Bus Selector2 : BusSelector  OutputSignals=Wheels.dZWheel,Wheels.omega,Driveline.WhlAng
  Constant1 : Constant  Value=zeros(4,1)  OutDataTypeStr=single
  Constant2 : Constant  Value=0  OutDataTypeStr=single
  Data Type Conversion{1,4..10,12} (9 alike) : DataTypeConversion  OutDataTypeStr=single
  Demux{,1..3} (4 alike) : Demux
  Integrator : Integrator  WrapState=on  WrappedStateUpperValue=2*pi  WrappedStateLowerValue=0  ZeroCross=off
  Part Rotation Concatenation : Subsystem
  Part Translation Concatenation : Subsystem
  Rate Transition : RateTransition  OutPortSampleTime=dt3D
  Scale : Subsystem
  Simulation 3D Engine 1 : sim3dlib/Simulation 3D Config  Priority=1  ProjectFormat=Executable  ProjectName=VehicleSimulation.exe  SceneDesc=Open surface  OpVisEn=off  Ts=dt3D  aMode=aMode
      settings: AttributesFormatString=Priority: %<Priority>  SourceProductName=Vehicle Dynamics Blockset  SourceProductBaseCode=VE
  Unary Minus : UnaryMinus
  Unary Minus1 : UnaryMinus
  Vehicle Actor Transform Set : sim3dlib/Simulation 3D Actor Transform Set  ActorTag=SimulinkVehicle1  ActorType=Passenger vehicle  PassVehMesh=Muscle car  VehColor=Red  NumberOfParts=5  CustNumOfParts=3  Translation=[X_o Y_o -Z_o; 0 0 0; 0 0 0; 0 0 0; 0 0 0]  Rotation=[phi_o theta_o psi_o; 0 0 0; 0 0 0; 0 0 0; 0 0 0]  Scale=[1 1 1; 1 1 1; 1 1 1; 1 1 1; 1 1 1]  Ts=dt3D  aMode=1
      settings: SourceProductName=Vehicle Dynamics Blockset  SourceProductBaseCode=VE
  VehicleActorTransform 2 : Subsystem  mask{depth=-5}
      mask prompts: depth "Initital Z position, depth (m):"
  wires:
  Unary Minus1/1 -> Data Type Conversion6/1
  Unary Minus/1 -> Integrator/1
  Bus Selector2/1 -> Data Type Conversion12/1  "<dZWheel>"
  Rate Transition/1 -> Bus Selector/1, Bus Selector2/1
  Scale/1(ScaleOut) -> Vehicle Actor Transform Set/3
  Demux/4 -> Part Rotation Concatenation/7(WheelRearRight Ptich)
  Demux/3 -> Part Rotation Concatenation/6(WheelRearLeft Pitch)
  Demux/2 -> Part Rotation Concatenation/5(WheelFrontRight Pitch)
  Demux/1 -> Part Rotation Concatenation/4(WheelFrontLeft Pitch)
  Constant1/1 -> Demux2/1
  Bus Selector/4 -> Data Type Conversion7/1  "<phi>"
  Part Rotation Concatenation/1(ConcatOut) -> Vehicle Actor Transform Set/2
  Part Translation Concatenation/1(ConcatOut) -> Vehicle Actor Transform Set/1
  Data Type Conversion12/1 -> Demux3/1
  Demux3/4 -> Part Translation Concatenation/15(WheelRearRightZ)
  Demux3/3 -> Part Translation Concatenation/14(WheelRearLeftZ)
  Demux3/1 -> Part Translation Concatenation/12(WheelFrontLeftZ)
  Demux3/2 -> Part Translation Concatenation/13(WheelFrontRightZ)
  VehFdbk/1 -> Rate Transition/1
  Data Type Conversion6/1 -> Part Translation Concatenation/3(BodyZ)
  Demux1/4 -> Part Rotation Concatenation/15(WheelRearRight Yaw)
  Demux1/3 -> Part Rotation Concatenation/14(WheelRearLeft Yaw)
  Demux2/1 -> Part Rotation Concatenation/8(WheelFrontLeft Roll)
  Demux2/2 -> Part Rotation Concatenation/9(WheelFrontRight Roll)
  Demux2/3 -> Part Rotation Concatenation/10(WheelRearLeft Roll)
  Demux2/4 -> Part Rotation Concatenation/11(WheelRearRight Roll)
  Bus Selector2/3 -> Data Type Conversion9/1  "<WhlAng>"
  Bus Selector2/2 -> Unary Minus/1  "<omega>"
  Data Type Conversion9/1 -> Demux1/1
  Demux1/1 -> Part Rotation Concatenation/12(WheelFrontLeft Yaw)
  Demux1/2 -> Part Rotation Concatenation/13(WheelFrontRight Yaw)
  Integrator/1 -> Data Type Conversion1/1
  Data Type Conversion1/1 -> Demux/1
  Data Type Conversion8/1 -> Part Rotation Concatenation/2(Body Ptich)
  Data Type Conversion5/1 -> Part Translation Concatenation/2(BodyY)
  Data Type Conversion10/1 -> Part Rotation Concatenation/3(Body Yaw)
  Constant2/1 -> Part Translation Concatenation/5(WheelFrontRightX), Part Translation Concatenation/6(WheelRearLeftX), Part Translation Concatenation/7(WheelRearRightX), Part Translation Concatenation/8(WheelFrontLeftY), Part Translation Concatenation/9(WheelFrontRightY), Part Translation Concatenation/10(WheelRearLeftY), Part Translation Concatenation/11(WheelRearRightY), Part Translation Concatenation/4(WheelFrontLeftX)
  Data Type Conversion4/1 -> Part Translation Concatenation/1(BodyX)
  Data Type Conversion7/1 -> Part Rotation Concatenation/1(Body Roll)
  Bus Selector/1 -> Data Type Conversion4/1  "<GeomX>"
  Bus Selector/2 -> Data Type Conversion5/1  "<GeomY>"
  Bus Selector/3 -> Unary Minus1/1  "<GeomZ>"
  Bus Selector/6 -> Data Type Conversion10/1  "<psi>"
  Bus Selector/5 -> Data Type Conversion8/1  "<theta>"

== system base_reference/Reference Generator/3D Engine/3D Engine Disabled ==
  VehFdbk : Inport
  Terminator : Terminator
  wires:
  VehFdbk/1 -> Terminator/1

== system base_reference/Reference Generator/Reference Generator/Constant Radius ==
  "VehFdbk " : Inport
  Bus Assignment : BusAssignment  AssignedSignals=Body.Y
  Bus Creator : BusCreator  Inputs=3
  Bus Creator1 : BusCreator  Inputs=4
  Bus Selector1 : BusSelector  OutputSignals=Body.ay
  Bus Selector2 : BusSelector  OutputSignals=Body.X,Body.Y,Body.psi,Body.Z
  Constant Radius : Subsystem  mask{Value=R, turnDirMask=Right}
      mask prompts: Value "Simulink:blkprm_prompts:ConstConstValue"; turnDirMask "Turn direction"
      mask TypeOptions Value: R/Value
      mask TypeOptions turnDirMask: Left | Right
      mask DialogControl Value Prompt: Constant value:
  Constant1 : Constant  Value=0
  Constant2 : Constant  Value=0
  Longitudinal Velocity Reference : Subsystem
  Signal Copy : SignalConversion  OverrideOpt=off
  ay Stop : vehdynlibscenariocommon/Slowly Increasing Steer/ay Stop  SystemSampleTime=-1
      settings: SourceProductName=Vehicle Dynamics Blockset  SourceProductBaseCode=VE
  " Vis" : Outport
  " Ref" : Outport  Port=2
  " Fdbk" : Outport  Port=3
  wires:
  Constant Radius/2(yFdbk) -> Bus Assignment/2
  Constant2/1 -> Bus Creator1/3  "Steer"
  Longitudinal Velocity Reference/1(xdot) -> Bus Creator1/1  "LngRef"
  Bus Creator1/1 -> " Ref"/1
  Constant1/1 -> Bus Creator1/4  "ThrotKill"
  Constant Radius/1(yRef) -> Bus Creator1/2  "LtrlRef"
  Bus Assignment/1 -> " Fdbk"/1
  Signal Copy/1 -> Bus Creator/3  "ZRef"
  Bus Creator/1 -> " Vis"/1
  Bus Selector2/4 -> Signal Copy/1  "<Z>"
  Constant Radius/4(YRef) -> Bus Creator/2  "YRef"
  "VehFdbk "/1 -> Bus Selector1/1, Bus Selector2/1, Bus Assignment/1
  Bus Selector2/2 -> Constant Radius/2(YVeh)  "<Y>"
  Bus Selector2/3 -> Constant Radius/3(psiVeh)  "<psi>"
  Bus Selector2/1 -> Constant Radius/1(XVeh)  "<X>"
  Constant Radius/3(XRef) -> Bus Creator/1  "XRef"
  Bus Selector1/1 -> ay Stop/1  "<ay>"

== system base_reference/Reference Generator/Reference Generator/Double Lane Change ==
  "VehFdbk " : Inport
  Double Lane Change : vehdynlibscenariocommon/Lane Change Reference Generator  VariantControl=Variant1  t_start=t_start  XGate=XGate  xdot_r=xdot_r  xdotUnit=mph  xStart=xStart  vehW=vehW  lattoff=lattoff  centerSwitch=on  latRefbp=latRefbp  latRef=latRef  aMode=2
      settings: SourceProductName=Vehicle Dynamics Blockset  SourceProductBaseCode=VE
  " Vis" : Outport
  " Ref" : Outport  Port=2
  " Fdbk" : Outport  Port=3
  wires:
  Double Lane Change/2 -> " Ref"/1
  Double Lane Change/1 -> " Vis"/1
  "VehFdbk "/1 -> Double Lane Change/1, " Fdbk"/1

== system base_reference/Reference Generator/Reference Generator/Increasing Steer ==
  "VehFdbk " : Inport
  Bus Creator : BusCreator  Inputs=3
  Ground : Ground
  Ground1 : Ground
  Ground2 : Ground
  Increasing Steer : vehdynlibscenariocommon/Slowly Increasing Steer  VariantControl=1  t_start=t_start  xdot_r=xdot_r  xdotUnit=mph  omega_hw=omega_hw  theta_max=theta_max  t_stop=t_stop  ay_max=ay_max  ay_stop=on  aMode=2
      settings: SourceProductName=Vehicle Dynamics Blockset  SourceProductBaseCode=VE
  " Vis" : Outport
  " Ref" : Outport  Port=2
  " Fdbk" : Outport  Port=3
  wires:
  Ground/1 -> Bus Creator/1  "XRef"
  Ground1/1 -> Bus Creator/2  "YRef"
  Ground2/1 -> Bus Creator/3  "ZRef"
  Increasing Steer/1 -> " Ref"/1  "LtrlRef"
  Bus Creator/1 -> " Vis"/1
  "VehFdbk "/1 -> Increasing Steer/1, " Fdbk"/1

== system base_reference/Reference Generator/Reference Generator/Sine with Dwell ==
  "VehFdbk " : Inport
  Bus Creator : BusCreator  Inputs=3
  Ground : Ground
  Ground1 : Ground
  Ground2 : Ground
  Sine With Dwell : vehdynlibscenariocommon/Sine With Dwell  VariantControl=3  t_start=t_start  xdot_r=xdot_r  xdotUnit=mph  steerF=steerF  steerA=steerA  tdwell=tdwell  steerDir=off  aMode=2
      settings: SourceProductName=Vehicle Dynamics Blockset  SourceProductBaseCode=VE
  " Vis" : Outport
  " Ref" : Outport  Port=2
  " Fdbk" : Outport  Port=3
  wires:
  Ground/1 -> Bus Creator/1  "XRef"
  Ground1/1 -> Bus Creator/2  "YRef"
  Ground2/1 -> Bus Creator/3  "ZRef"
  Bus Creator/1 -> " Vis"/1
  "VehFdbk "/1 -> Sine With Dwell/1, " Fdbk"/1
  Sine With Dwell/1 -> " Ref"/1

== system base_reference/Reference Generator/Reference Generator/Swept Sine ==
  "VehFdbk " : Inport
  Bus Creator : BusCreator  Inputs=3
  Ground : Ground
  Ground1 : Ground
  Ground2 : Ground
  Swept Sine : vehdynlibscenariocommon/Swept Sine Reference Generator  VariantControl=2  t_start=t_start  xdot_r=xdot_r  xdotUnit=mph  theta_hw=theta_hw  theta_hw_final=theta_hw_final  t_sweep=t_sweep  aMode=2
      settings: SourceProductName=Vehicle Dynamics Blockset  SourceProductBaseCode=VE
  " Vis" : Outport
  " Ref" : Outport  Port=2
  " Fdbk" : Outport  Port=3
  wires:
  Ground/1 -> Bus Creator/1  "XRef"
  Ground1/1 -> Bus Creator/2  "YRef"
  Ground2/1 -> Bus Creator/3  "ZRef"
  Bus Creator/1 -> " Vis"/1
  Swept Sine/1 -> " Ref"/1
  "VehFdbk "/1 -> Swept Sine/1, " Fdbk"/1

== system base_reference/Visualization/ISO 15037-1:2006/Disabled ==
  VehFdbk : Inport
  Cntrl : Inport  Port=2
  Terminator : Terminator
  Terminator1 : Terminator
  wires:
  Cntrl/1 -> Terminator/1
  VehFdbk/1 -> Terminator1/1
